simulink model "magball_linear_older_ver"  (R2022a)
settings: Solver=VariableStepAuto  StartTime=0.0  StopTime=2  RelTol=1e-3
undefined symbols (not defined in the file): A1, B1, C1, D1, i0, y0
settings Model: Creator=xiaom  LastModifiedBy=cr
settings ModelReferenceCC: EnableRefExpFcnMdlSchedulingChecks=off
settings RTWCC: Description=Generic Real-Time Target

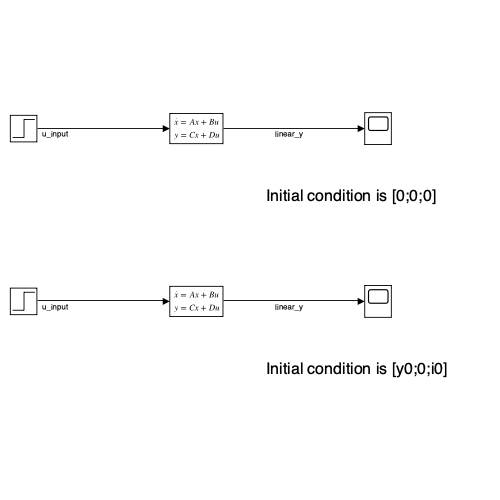
[thumbnail: Simulink's stored preview of the top-level diagram]
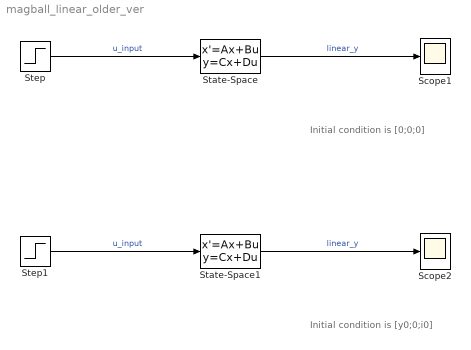
== system magball_linear_older_ver ==
  note: Initial condition is [0;0;0]
  note: Initial condition is [y0;0;i0]
  Scope1 : Scope
  Scope2 : Scope
  State-Space : StateSpace  A=A1  B=B1  C=C1  D=D1  InitialCondition=[0,0,0]
  State-Space1 : StateSpace  A=A1  B=B1  C=C1  D=D1  InitialCondition=[y0;0;i0]
  Step : Step  Time=0  SampleTime=0
  Step1 : Step  Time=0  SampleTime=0
  wires:
  State-Space/1 -> Scope1/1  "linear_y"
  Step/1 -> State-Space/1  "u_input"
  Step1/1 -> State-Space1/1  "u_input"
  State-Space1/1 -> Scope2/1  "linear_y"
